simulink model "FCSFunctional"  (R2025b)
settings: Solver=VariableStepAuto  StartTime=0.0  StopTime=10.0  RelTol=1e-3
settings Model: DataDictionary=FCSInterfaces.sldd  Creator=sarah  LastModifiedBy=sarah

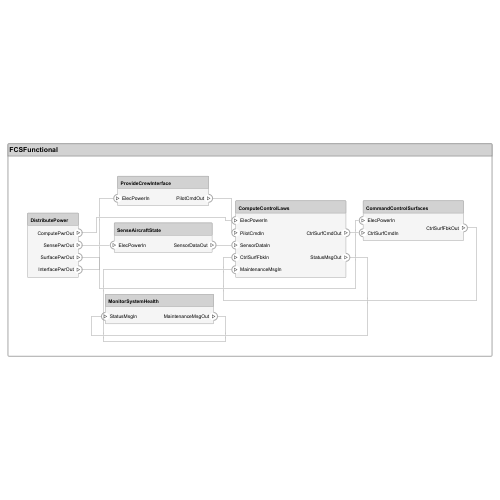
[thumbnail: Simulink's stored preview of the top-level diagram]
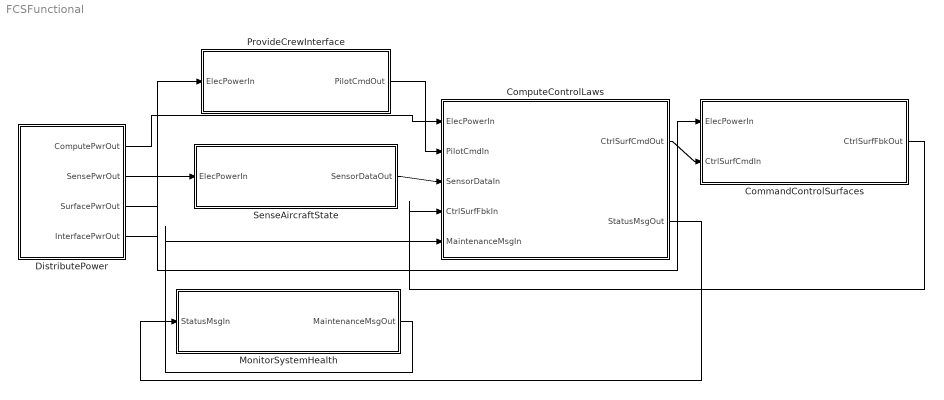
== system FCSFunctional ==
  CommandControlSurfaces : Subsystem
      settings: PortSchema="{\"entries\":[{\"content\":{\"headerSize\":26,\"margin\":15,\"minimumSpacing\":25,\"sides\":[{\"content\":{\"connectorIds\":[\"In1\",\"In2\"]},\"type\":\"ConnectorPlacement.EquallySpacedRectSide\",\"uuid\":\"20d6bed0-d8e5-4088-8794-9345a2942e90\"},{\"content\":{\"connectorIds\":[\"Out1\"],\"side\":\"RIGHT\"},\"type\":\"ConnectorPlacement.EquallySpacedRectSide\",\"uuid\":\"e7adde65-1579-42e2-b600-0f533305a23b\"},{\"content\":{\"side\":\"TOP\"},\"type\":\"ConnectorPlacement.EquallySpacedRectSide\",\"uuid\":\"73636ec6-6908-4b74-b302-6e84b019a70e\"}]},\"type\":\"ConnectorPlacement.EquallySpacedConnector\",\"uuid\":\"cc5d9ea4-0f09-4026-9dcf-92b706ac45bf\"}],\"packageUris\":[\"http://schema.mathworks.com/mf0/Connector/R2020b\"],\"version\":\"1.0\"}"
  ComputeControlLaws : Subsystem
      settings: PortSchema="{\"entries\":[{\"content\":{\"headerSize\":26,\"margin\":15,\"minimumSpacing\":25,\"sides\":[{\"content\":{\"connectorIds\":[\"In1\",\"In2\",\"In3\",\"In4\",\"In5\"]},\"type\":\"ConnectorPlacement.EquallySpacedRectSide\",\"uuid\":\"20d6bed0-d8e5-4088-8794-9345a2942e90\"},{\"content\":{\"connectorIds\":[\"Out1\",\"Out2\"],\"side\":\"RIGHT\"},\"type\":\"ConnectorPlacement.EquallySpacedRectSide\",\"uuid\":\"e7adde65-1579-42e2-b600-0f533305a23b\"},{\"content\":{\"side\":\"TOP\"},\"type\":\"ConnectorPlacement.EquallySpacedRectSide\",\"uuid\":\"73636ec6-6908-4b74-b302-6e84b019a70e\"}]},\"type\":\"ConnectorPlacement.EquallySpacedConnector\",\"uuid\":\"cc5d9ea4-0f09-4026-9dcf-92b706ac45bf\"}],\"packageUris\":[\"http://schema.mathworks.com/mf0/Connector/R2020b\"],\"version\":\"1.0\"}"
  DistributePower : Subsystem
      settings: PortSchema="{\"entries\":[{\"content\":{\"headerSize\":26,\"margin\":15,\"minimumSpacing\":25,\"sides\":[{\"content\":{},\"type\":\"ConnectorPlacement.EquallySpacedRectSide\",\"uuid\":\"20d6bed0-d8e5-4088-8794-9345a2942e90\"},{\"content\":{\"connectorIds\":[\"Out1\",\"Out2\",\"Out3\",\"Out4\"],\"side\":\"RIGHT\"},\"type\":\"ConnectorPlacement.EquallySpacedRectSide\",\"uuid\":\"e7adde65-1579-42e2-b600-0f533305a23b\"},{\"content\":{\"side\":\"TOP\"},\"type\":\"ConnectorPlacement.EquallySpacedRectSide\",\"uuid\":\"73636ec6-6908-4b74-b302-6e84b019a70e\"}]},\"type\":\"ConnectorPlacement.EquallySpacedConnector\",\"uuid\":\"cc5d9ea4-0f09-4026-9dcf-92b706ac45bf\"}],\"packageUris\":[\"http://schema.mathworks.com/mf0/Connector/R2020b\"],\"version\":\"1.0\"}"
  MonitorSystemHealth : Subsystem
      settings: PortSchema="{\"entries\":[{\"content\":{\"headerSize\":26,\"margin\":15,\"minimumSpacing\":25,\"sides\":[{\"content\":{\"connectorIds\":[\"In1\"]},\"type\":\"ConnectorPlacement.EquallySpacedRectSide\",\"uuid\":\"20d6bed0-d8e5-4088-8794-9345a2942e90\"},{\"content\":{\"connectorIds\":[\"Out1\"],\"side\":\"RIGHT\"},\"type\":\"ConnectorPlacement.EquallySpacedRectSide\",\"uuid\":\"e7adde65-1579-42e2-b600-0f533305a23b\"},{\"content\":{\"side\":\"TOP\"},\"type\":\"ConnectorPlacement.EquallySpacedRectSide\",\"uuid\":\"73636ec6-6908-4b74-b302-6e84b019a70e\"}]},\"type\":\"ConnectorPlacement.EquallySpacedConnector\",\"uuid\":\"cc5d9ea4-0f09-4026-9dcf-92b706ac45bf\"}],\"packageUris\":[\"http://schema.mathworks.com/mf0/Connector/R2020b\"],\"version\":\"1.0\"}"
  ProvideCrewInterface : Subsystem
      settings: PortSchema="{\"entries\":[{\"content\":{\"headerSize\":26,\"margin\":15,\"minimumSpacing\":25,\"sides\":[{\"content\":{\"connectorIds\":[\"In1\"]},\"type\":\"ConnectorPlacement.EquallySpacedRectSide\",\"uuid\":\"20d6bed0-d8e5-4088-8794-9345a2942e90\"},{\"content\":{\"connectorIds\":[\"Out1\"],\"side\":\"RIGHT\"},\"type\":\"ConnectorPlacement.EquallySpacedRectSide\",\"uuid\":\"e7adde65-1579-42e2-b600-0f533305a23b\"},{\"content\":{\"side\":\"TOP\"},\"type\":\"ConnectorPlacement.EquallySpacedRectSide\",\"uuid\":\"73636ec6-6908-4b74-b302-6e84b019a70e\"}]},\"type\":\"ConnectorPlacement.EquallySpacedConnector\",\"uuid\":\"cc5d9ea4-0f09-4026-9dcf-92b706ac45bf\"}],\"packageUris\":[\"http://schema.mathworks.com/mf0/Connector/R2020b\"],\"version\":\"1.0\"}"
  SenseAircraftState : Subsystem
      settings: PortSchema="{\"entries\":[{\"content\":{\"headerSize\":26,\"margin\":15,\"minimumSpacing\":25,\"sides\":[{\"content\":{\"connectorIds\":[\"In1\"]},\"type\":\"ConnectorPlacement.EquallySpacedRectSide\",\"uuid\":\"20d6bed0-d8e5-4088-8794-9345a2942e90\"},{\"content\":{\"connectorIds\":[\"Out1\"],\"side\":\"RIGHT\"},\"type\":\"ConnectorPlacement.EquallySpacedRectSide\",\"uuid\":\"e7adde65-1579-42e2-b600-0f533305a23b\"},{\"content\":{\"side\":\"TOP\"},\"type\":\"ConnectorPlacement.EquallySpacedRectSide\",\"uuid\":\"73636ec6-6908-4b74-b302-6e84b019a70e\"}]},\"type\":\"ConnectorPlacement.EquallySpacedConnector\",\"uuid\":\"cc5d9ea4-0f09-4026-9dcf-92b706ac45bf\"}],\"packageUris\":[\"http://schema.mathworks.com/mf0/Connector/R2020b\"],\"version\":\"1.0\"}"
  wires:
  DistributePower/2(SensePwrOut) -> SenseAircraftState/1(ElecPowerIn)
  DistributePower/1(ComputePwrOut) -> ComputeControlLaws/1(ElecPowerIn)
  DistributePower/3(SurfacePwrOut) -> CommandControlSurfaces/1(ElecPowerIn)
  ComputeControlLaws/1(CtrlSurfCmdOut) -> CommandControlSurfaces/2(CtrlSurfCmdIn)
  ComputeControlLaws/2(StatusMsgOut) -> MonitorSystemHealth/1(StatusMsgIn)
  MonitorSystemHealth/1(MaintenanceMsgOut) -> ComputeControlLaws/5(MaintenanceMsgIn)
  DistributePower/4(InterfacePwrOut) -> ProvideCrewInterface/1(ElecPowerIn)
  ProvideCrewInterface/1(PilotCmdOut) -> ComputeControlLaws/2(PilotCmdIn)
  SenseAircraftState/1(SensorDataOut) -> ComputeControlLaws/3(SensorDataIn)
  CommandControlSurfaces/1(CtrlSurfFbkOut) -> ComputeControlLaws/4(CtrlSurfFbkIn)

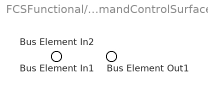
== system FCSFunctional/CommandControlSurfaces ==
  Bus Element In1 : Inport  PortName=ElecPowerIn
  Bus Element In2 : Inport  Port=2  PortName=CtrlSurfCmdIn
  Bus Element Out1 : Outport  PortName=CtrlSurfFbkOut

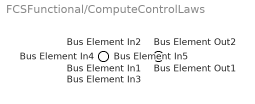
== system FCSFunctional/ComputeControlLaws ==
  Bus Element In1 : Inport  PortName=ElecPowerIn
  Bus Element In2 : Inport  Port=2  PortName=PilotCmdIn
  Bus Element In3 : Inport  Port=3  PortName=SensorDataIn
  Bus Element In4 : Inport  Port=4  PortName=CtrlSurfFbkIn
  Bus Element In5 : Inport  Port=5  PortName=MaintenanceMsgIn
  Bus Element Out1 : Outport  PortName=CtrlSurfCmdOut
  Bus Element Out2 : Outport  Port=2  PortName=StatusMsgOut

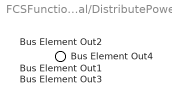
== system FCSFunctional/DistributePower ==
  Bus Element Out1 : Outport  PortName=ComputePwrOut
  Bus Element Out2 : Outport  Port=2  PortName=SensePwrOut
  Bus Element Out3 : Outport  Port=3  PortName=SurfacePwrOut
  Bus Element Out4 : Outport  Port=4  PortName=InterfacePwrOut

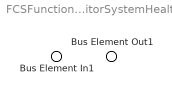
== system FCSFunctional/MonitorSystemHealth ==
  Bus Element In1 : Inport  PortName=StatusMsgIn
  Bus Element Out1 : Outport  PortName=MaintenanceMsgOut

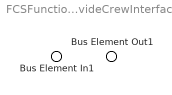
== system FCSFunctional/ProvideCrewInterface ==
  Bus Element In1 : Inport  PortName=ElecPowerIn
  Bus Element Out1 : Outport  PortName=PilotCmdOut

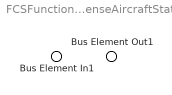
== system FCSFunctional/SenseAircraftState ==
  Bus Element In1 : Inport  PortName=ElecPowerIn
  Bus Element Out1 : Outport  PortName=SensorDataOut
